simulink model "All_Controller_Compare"  (R2022a)
settings: Solver=VariableStepAuto  StartTime=0.0  StopTime=12.5  RelTol=1e-3
undefined symbols (not defined in the file): A, att_opt, B, C, ki_u4_, Klqr, L, pitch_opt, roll_opt, x_opt, y_opt, yaw_opt
libraries: slpidlib x6
settings Model: Creator=creec  LastModifiedBy=creec

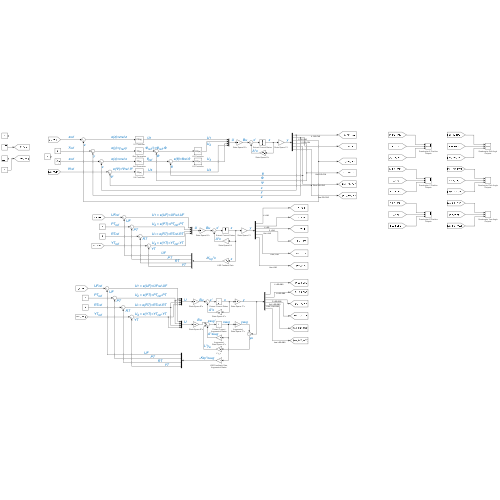
[thumbnail: Simulink's stored preview of the top-level diagram]
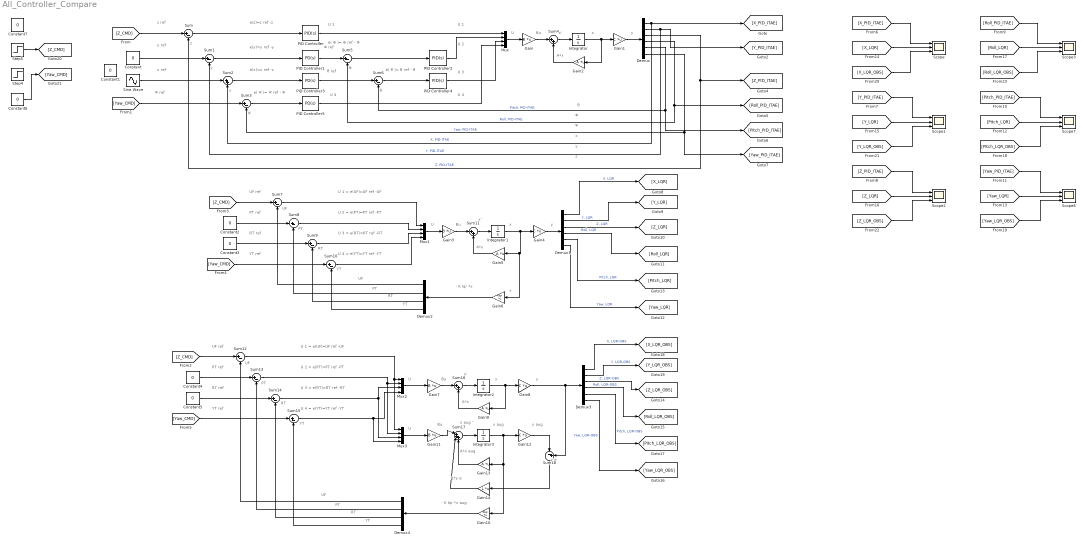
== system All_Controller_Compare ==
  note: z
  note: x ref
  note: U 1
  note: U 4
  note: x
  note: Ψ
  note: x'
  note: θ
  note: Ψ ref
  note: e(y)=y ref -y
  note: e(x)=x ref -x
  note: U 1
  note: e( θ )= θ ref - θ
  note: Φ ref
  note: x
  note: x
  note: Ψ
  note: A*x
  note: e(z)=z ref -z
  note: y
  note: U 2
  note: U
  note: z
  note: θ
  note: Bu
  note: U 4
  note: Φ
  note: Φ
  note: y ref
  note: y
  note: y
  note: z ref
  note: e( Ψ )= Ψ ref - Ψ
  note: U 3
  note: θ ref
  note: e( Φ )= Φ ref - Φ
  note: PT
  note: y
  note: U 3 = e(RT)=RT ref -RT
  note: U 4 = e(YT)=YT ref -YT
  note: U 2 = e(PT)=PT ref -PT
  note: x
  note: RT
  note: PT
  note: - K lqr *x
  note: UF
  note: Bu
  note: UF ref
  note: U 1 = e(UF)=UF ref -UF
  note: RT ref
  note: x
  note: UF
  note: A*x
  note: YT ref
  note: PT ref
  note: U
  note: x'
  note: YT
  note: RT
  note: YT
  note: x aug
  note: L*y e
  note: RT ref
  note: YT ref
  note: x
  note: U
  note: YT
  note: U 1 = e(UF)=UF ref -UF
  note: x'
  note: A*x
  note: YT
  note: A*x aug
  note: PT ref
  note: UF
  note: U
  note: UF
  note: UF ref
  note: Bu
  note: RT
  note: U 2 = e(PT)=PT ref -PT
  note: RT
  note: U 4 = e(YT)=YT ref -YT
  note: x aug '
  note: PT
  note: U 3 = e(RT)=RT ref -RT
  note: PT
  note: y e
  note: - K lqr *x aug
  note: y
  note: y aug
  note: Bu
  Constant{,1..7} (8 alike) : Constant  Value=0
  Demux : Demux  Outputs=6
  Demux1 : Demux  Outputs=6
  Demux2 : Demux
  Demux3 : Demux  Outputs=6
  Demux4 : Demux
  Gain{,3,7,11} (4 alike) : Gain  Gain=B  Multiplication=Matrix(K*u)
      settings: AttributesFormatString=State-Space B*u
  Gain{1,4,8,12} (4 alike) : Gain  Gain=C  Multiplication=Matrix(K*u)
      Gain1 settings: AttributesFormatString=State-Space C*x
      Gain12 settings: AttributesFormatString=|
      | Augmented
      | State-Space C*x
      Gain4 settings: AttributesFormatString=State-Space C*x
      Gain8 settings: AttributesFormatString=State-Space C*x
  Gain10 : Gain  Gain=Klqr  Multiplication=Matrix(K*u)
      settings: AttributesFormatString=|
      | LQR Feedback Gain,
      | Augmented States
  Gain{2,5,9,13} (4 alike) : Gain  Gain=A  Multiplication=Matrix(K*u)
      Gain13 settings: AttributesFormatString=|
      | Augmented
      | State-Space A*x
      Gain2 settings: AttributesFormatString=State-Space A*x
      Gain5 settings: AttributesFormatString=State-Space A*x
      Gain9 settings: AttributesFormatString=State-Space A*x
  Gain14 : Gain  Gain=L  Multiplication=Matrix(K*u)
      settings: AttributesFormatString=L*y_e
  Gain6 : Gain  Gain=Klqr  Multiplication=Matrix(K*u)
      settings: AttributesFormatString=LQR Feeback Gain
  Integrator{,1..3} (4 alike) : Integrator
      Integrator settings: AttributesFormatString=Extract Current States
      Integrator1 settings: AttributesFormatString=Extract Current States
      Integrator2 settings: AttributesFormatString=Extract Current States
      Integrator3 settings: AttributesFormatString=|
      | Extract Current
      | Augmented States
  Mux{,1..3} (4 alike) : Mux
  PID Controller : slpidlib/PID Controller  Controller=PID  Form=Parallel  TimeDomain=Continuous-time  UseExternalTs=off  SampleTime=-1  IntegratorMethod=Forward Euler  FilterMethod=Forward Euler  ControllerParametersSource=internal  P=att_opt(1)  I=att_opt(2)  UseKiTs=off  D=att_opt(3)  N=100  UseFilter=on  TunerSelectOption=Transfer Function Based (PID Tuner App)  InitialConditionSource=internal  InitialConditionForIntegrator=0  InitialConditionForFilter=0  DifferentiatorICPrevScaledInput=0  ExternalReset=none  TrackingMode=off  Kt=1  LimitOutput=off  SatLimitsSource=internal  UpperSaturationLimit=inf  LowerSaturationLimit=-inf  LinearizeAsGain=on  AntiWindupMode=none  Kb=1  POutMin=[]  POutMax=[]  IOutMin=[]  IOutMax=[]  DOutMin=[]  DOutMax=[]  NOutMin=[]  NOutMax=[]  SumOutMin=[]  SumOutMax=[]  SaturationOutMin=[]  SaturationOutMax=[]  PParamMin=[]  PParamMax=[]  IParamMin=[]  IParamMax=[]  DParamMin=[]  DParamMax=[]  NParamMin=[]  NParamMax=[]  KbParamMin=[]  KbParamMax=[]  KtParamMin=[]  KtParamMax=[]  KbOutMin=[]  KbOutMax=[]  KtOutMin=[]  KtOutMax=[]  IntegratorOutMin=[]  IntegratorOutMax=[]  FilterOutMin=[]  FilterOutMax=[]  SumI1OutMin=[]  SumI1OutMax=[]  SumI2OutMin=[]  SumI2OutMax=[]  SumI3OutMin=[]  SumI3OutMax=[]  SumI4OutMin=[]  SumI4OutMax=[]  SumDOutMin=[]  SumDOutMax=[]  DifferentiatorOutMin=[]  DifferentiatorOutMax=[]  FilterDiffOutCoefMin=[]  FilterDiffOutCoefMax=[]  ReciprocalOutMin=[]  ReciprocalOutMax=[]  SumDenOutMin=[]  SumDenOutMax=[]  SumNumOutMin=[]  SumNumOutMax=[]  DivideOutMin=[]  DivideOutMax=[]  UdiffTsProdOutMin=[]  UdiffTsProdOutMax=[]  NTsProdOutMin=[]  NTsProdOutMax=[]  UintegralTsProdOutMin=[]  UintegralTsProdOutMax=[]  UngainTsProdOutMin=[]  UngainTsProdOutMax=[]  IntegratorContinuousStateAttributes=''  IntegratorStateMustResolveToSignalObject=off  IntegratorRTWStateStorageClass=Auto  FilterContinuousStateAttributes=''  FilterStateMustResolveToSignalObject=off  FilterRTWStateStorageClass=Auto  ParallelPVariant=InternalParameters  IdealPVariant=Disabled  IVariant=InternalParameters  DVariant=InternalParameters  IntegratorVariant=Continuous  SatVariant=Disabled  AWVariant=Passthrough  PCopyVariant=Disabled  TRVariant=Disabled  FdbkBlocksVariant=Forward  IdealPFdbkVariant=Disabled  SatFdbkVariant=Disabled  DerivativeFilterVariant=ContFilter  NVariant=InternalParameters  NCopyVariant=Disabled  FilterICVariant=InternalICsFilter  IntegratorICVariant=InternalICs  ExternalResetVariant=Disabled  TRSumVariant=Passthrough  SumFdbkVariant=Disabled  SumVariant=Sum_PID  TsampFilterVariant=InternalTs  TsampNgainVariant=Passthrough  TsampIntegralVariant=Passthrough  ExternalSaturationOutDataTypeStr=Inherit: Same as second input  aMode=0
      settings: AttributesFormatString=U1 Controller
  PID Controller1 : slpidlib/PID Controller  Controller=PD  Form=Parallel  TimeDomain=Continuous-time  UseExternalTs=off  SampleTime=-1  IntegratorMethod=Forward Euler  FilterMethod=Forward Euler  ControllerParametersSource=internal  P=y_opt(1)  I=0  UseKiTs=off  D=y_opt(2)  N=100  UseFilter=on  TunerSelectOption=Transfer Function Based (PID Tuner App)  InitialConditionSource=internal  InitialConditionForIntegrator=0  InitialConditionForFilter=0  DifferentiatorICPrevScaledInput=0  ExternalReset=none  TrackingMode=off  Kt=1  LimitOutput=off  SatLimitsSource=internal  UpperSaturationLimit=inf  LowerSaturationLimit=-inf  LinearizeAsGain=on  AntiWindupMode=none  Kb=1  POutMin=[]  POutMax=[]  IOutMin=[]  IOutMax=[]  DOutMin=[]  DOutMax=[]  NOutMin=[]  NOutMax=[]  SumOutMin=[]  SumOutMax=[]  SaturationOutMin=[]  SaturationOutMax=[]  PParamMin=[]  PParamMax=[]  IParamMin=[]  IParamMax=[]  DParamMin=[]  DParamMax=[]  NParamMin=[]  NParamMax=[]  KbParamMin=[]  KbParamMax=[]  KtParamMin=[]  KtParamMax=[]  KbOutMin=[]  KbOutMax=[]  KtOutMin=[]  KtOutMax=[]  IntegratorOutMin=[]  IntegratorOutMax=[]  FilterOutMin=[]  FilterOutMax=[]  SumI1OutMin=[]  SumI1OutMax=[]  SumI2OutMin=[]  SumI2OutMax=[]  SumI3OutMin=[]  SumI3OutMax=[]  SumI4OutMin=[]  SumI4OutMax=[]  SumDOutMin=[]  SumDOutMax=[]  DifferentiatorOutMin=[]  DifferentiatorOutMax=[]  FilterDiffOutCoefMin=[]  FilterDiffOutCoefMax=[]  ReciprocalOutMin=[]  ReciprocalOutMax=[]  SumDenOutMin=[]  SumDenOutMax=[]  SumNumOutMin=[]  SumNumOutMax=[]  DivideOutMin=[]  DivideOutMax=[]  UdiffTsProdOutMin=[]  UdiffTsProdOutMax=[]  NTsProdOutMin=[]  NTsProdOutMax=[]  UintegralTsProdOutMin=[]  UintegralTsProdOutMax=[]  UngainTsProdOutMin=[]  UngainTsProdOutMax=[]  IntegratorContinuousStateAttributes=''  IntegratorStateMustResolveToSignalObject=off  IntegratorRTWStateStorageClass=Auto  FilterContinuousStateAttributes=''  FilterStateMustResolveToSignalObject=off  FilterRTWStateStorageClass=Auto  ParallelPVariant=InternalParameters  IdealPVariant=Disabled  IVariant=Disabled  DVariant=InternalParameters  IntegratorVariant=Disabled  SatVariant=Disabled  AWVariant=Disabled  PCopyVariant=Disabled  TRVariant=Disabled  FdbkBlocksVariant=Forward  IdealPFdbkVariant=Disabled  SatFdbkVariant=Disabled  DerivativeFilterVariant=ContFilter  NVariant=InternalParameters  NCopyVariant=Disabled  FilterICVariant=InternalICsFilter  IntegratorICVariant=Disabled  ExternalResetVariant=Disabled  TRSumVariant=Passthrough  SumFdbkVariant=Disabled  SumVariant=Sum_PD  TsampFilterVariant=InternalTs  TsampNgainVariant=Passthrough  TsampIntegralVariant=Disabled_SignalSpec  ExternalSaturationOutDataTypeStr=Inherit: Same as second input  aMode=0
      settings: AttributesFormatString=Φref Generation
  PID Controller2 : slpidlib/PID Controller  Controller=PID  Form=Parallel  TimeDomain=Continuous-time  UseExternalTs=off  SampleTime=-1  IntegratorMethod=Forward Euler  FilterMethod=Forward Euler  ControllerParametersSource=internal  P=pitch_opt(1)  I=pitch_opt(2)  UseKiTs=off  D=pitch_opt(3)  N=100  UseFilter=on  TunerSelectOption=Transfer Function Based (PID Tuner App)  InitialConditionSource=internal  InitialConditionForIntegrator=0  InitialConditionForFilter=0  DifferentiatorICPrevScaledInput=0  ExternalReset=none  TrackingMode=off  Kt=1  LimitOutput=off  SatLimitsSource=internal  UpperSaturationLimit=inf  LowerSaturationLimit=-inf  LinearizeAsGain=on  AntiWindupMode=none  Kb=1  POutMin=[]  POutMax=[]  IOutMin=[]  IOutMax=[]  DOutMin=[]  DOutMax=[]  NOutMin=[]  NOutMax=[]  SumOutMin=[]  SumOutMax=[]  SaturationOutMin=[]  SaturationOutMax=[]  PParamMin=[]  PParamMax=[]  IParamMin=[]  IParamMax=[]  DParamMin=[]  DParamMax=[]  NParamMin=[]  NParamMax=[]  KbParamMin=[]  KbParamMax=[]  KtParamMin=[]  KtParamMax=[]  KbOutMin=[]  KbOutMax=[]  KtOutMin=[]  KtOutMax=[]  IntegratorOutMin=[]  IntegratorOutMax=[]  FilterOutMin=[]  FilterOutMax=[]  SumI1OutMin=[]  SumI1OutMax=[]  SumI2OutMin=[]  SumI2OutMax=[]  SumI3OutMin=[]  SumI3OutMax=[]  SumI4OutMin=[]  SumI4OutMax=[]  SumDOutMin=[]  SumDOutMax=[]  DifferentiatorOutMin=[]  DifferentiatorOutMax=[]  FilterDiffOutCoefMin=[]  FilterDiffOutCoefMax=[]  ReciprocalOutMin=[]  ReciprocalOutMax=[]  SumDenOutMin=[]  SumDenOutMax=[]  SumNumOutMin=[]  SumNumOutMax=[]  DivideOutMin=[]  DivideOutMax=[]  UdiffTsProdOutMin=[]  UdiffTsProdOutMax=[]  NTsProdOutMin=[]  NTsProdOutMax=[]  UintegralTsProdOutMin=[]  UintegralTsProdOutMax=[]  UngainTsProdOutMin=[]  UngainTsProdOutMax=[]  IntegratorContinuousStateAttributes=''  IntegratorStateMustResolveToSignalObject=off  IntegratorRTWStateStorageClass=Auto  FilterContinuousStateAttributes=''  FilterStateMustResolveToSignalObject=off  FilterRTWStateStorageClass=Auto  ParallelPVariant=InternalParameters  IdealPVariant=Disabled  IVariant=InternalParameters  DVariant=InternalParameters  IntegratorVariant=Continuous  SatVariant=Disabled  AWVariant=Passthrough  PCopyVariant=Disabled  TRVariant=Disabled  FdbkBlocksVariant=Forward  IdealPFdbkVariant=Disabled  SatFdbkVariant=Disabled  DerivativeFilterVariant=ContFilter  NVariant=InternalParameters  NCopyVariant=Disabled  FilterICVariant=InternalICsFilter  IntegratorICVariant=InternalICs  ExternalResetVariant=Disabled  TRSumVariant=Passthrough  SumFdbkVariant=Disabled  SumVariant=Sum_PID  TsampFilterVariant=InternalTs  TsampNgainVariant=Passthrough  TsampIntegralVariant=Passthrough  ExternalSaturationOutDataTypeStr=Inherit: Same as second input  aMode=0
      settings: AttributesFormatString=U2 Controller
  PID Controller3 : slpidlib/PID Controller  Controller=PD  Form=Parallel  TimeDomain=Continuous-time  UseExternalTs=off  SampleTime=-1  IntegratorMethod=Forward Euler  FilterMethod=Forward Euler  ControllerParametersSource=internal  P=x_opt(1)  I=-0.0096  UseKiTs=off  D=x_opt(2)  N=100  UseFilter=on  TunerSelectOption=Transfer Function Based (PID Tuner App)  InitialConditionSource=internal  InitialConditionForIntegrator=0  InitialConditionForFilter=0  DifferentiatorICPrevScaledInput=0  ExternalReset=none  TrackingMode=off  Kt=1  LimitOutput=off  SatLimitsSource=internal  UpperSaturationLimit=inf  LowerSaturationLimit=-inf  LinearizeAsGain=on  AntiWindupMode=none  Kb=1  POutMin=[]  POutMax=[]  IOutMin=[]  IOutMax=[]  DOutMin=[]  DOutMax=[]  NOutMin=[]  NOutMax=[]  SumOutMin=[]  SumOutMax=[]  SaturationOutMin=[]  SaturationOutMax=[]  PParamMin=[]  PParamMax=[]  IParamMin=[]  IParamMax=[]  DParamMin=[]  DParamMax=[]  NParamMin=[]  NParamMax=[]  KbParamMin=[]  KbParamMax=[]  KtParamMin=[]  KtParamMax=[]  KbOutMin=[]  KbOutMax=[]  KtOutMin=[]  KtOutMax=[]  IntegratorOutMin=[]  IntegratorOutMax=[]  FilterOutMin=[]  FilterOutMax=[]  SumI1OutMin=[]  SumI1OutMax=[]  SumI2OutMin=[]  SumI2OutMax=[]  SumI3OutMin=[]  SumI3OutMax=[]  SumI4OutMin=[]  SumI4OutMax=[]  SumDOutMin=[]  SumDOutMax=[]  DifferentiatorOutMin=[]  DifferentiatorOutMax=[]  FilterDiffOutCoefMin=[]  FilterDiffOutCoefMax=[]  ReciprocalOutMin=[]  ReciprocalOutMax=[]  SumDenOutMin=[]  SumDenOutMax=[]  SumNumOutMin=[]  SumNumOutMax=[]  DivideOutMin=[]  DivideOutMax=[]  UdiffTsProdOutMin=[]  UdiffTsProdOutMax=[]  NTsProdOutMin=[]  NTsProdOutMax=[]  UintegralTsProdOutMin=[]  UintegralTsProdOutMax=[]  UngainTsProdOutMin=[]  UngainTsProdOutMax=[]  IntegratorContinuousStateAttributes=''  IntegratorStateMustResolveToSignalObject=off  IntegratorRTWStateStorageClass=Auto  FilterContinuousStateAttributes=''  FilterStateMustResolveToSignalObject=off  FilterRTWStateStorageClass=Auto  ParallelPVariant=InternalParameters  IdealPVariant=Disabled  IVariant=Disabled  DVariant=InternalParameters  IntegratorVariant=Disabled  SatVariant=Disabled  AWVariant=Disabled  PCopyVariant=Disabled  TRVariant=Disabled  FdbkBlocksVariant=Forward  IdealPFdbkVariant=Disabled  SatFdbkVariant=Disabled  DerivativeFilterVariant=ContFilter  NVariant=InternalParameters  NCopyVariant=Disabled  FilterICVariant=InternalICsFilter  IntegratorICVariant=Disabled  ExternalResetVariant=Disabled  TRSumVariant=Passthrough  SumFdbkVariant=Disabled  SumVariant=Sum_PD  TsampFilterVariant=InternalTs  TsampNgainVariant=Passthrough  TsampIntegralVariant=Disabled_SignalSpec  ExternalSaturationOutDataTypeStr=Inherit: Same as second input  aMode=0
      settings: AttributesFormatString=θref Generation
  PID Controller4 : slpidlib/PID Controller  Controller=PID  Form=Parallel  TimeDomain=Continuous-time  UseExternalTs=off  SampleTime=-1  IntegratorMethod=Forward Euler  FilterMethod=Forward Euler  ControllerParametersSource=internal  P=roll_opt(1)  I=roll_opt(2)  UseKiTs=off  D=roll_opt(3)  N=100  UseFilter=on  TunerSelectOption=Transfer Function Based (PID Tuner App)  InitialConditionSource=internal  InitialConditionForIntegrator=0  InitialConditionForFilter=0  DifferentiatorICPrevScaledInput=0  ExternalReset=none  TrackingMode=off  Kt=1  LimitOutput=off  SatLimitsSource=internal  UpperSaturationLimit=inf  LowerSaturationLimit=-inf  LinearizeAsGain=on  AntiWindupMode=none  Kb=1  POutMin=[]  POutMax=[]  IOutMin=[]  IOutMax=[]  DOutMin=[]  DOutMax=[]  NOutMin=[]  NOutMax=[]  SumOutMin=[]  SumOutMax=[]  SaturationOutMin=[]  SaturationOutMax=[]  PParamMin=[]  PParamMax=[]  IParamMin=[]  IParamMax=[]  DParamMin=[]  DParamMax=[]  NParamMin=[]  NParamMax=[]  KbParamMin=[]  KbParamMax=[]  KtParamMin=[]  KtParamMax=[]  KbOutMin=[]  KbOutMax=[]  KtOutMin=[]  KtOutMax=[]  IntegratorOutMin=[]  IntegratorOutMax=[]  FilterOutMin=[]  FilterOutMax=[]  SumI1OutMin=[]  SumI1OutMax=[]  SumI2OutMin=[]  SumI2OutMax=[]  SumI3OutMin=[]  SumI3OutMax=[]  SumI4OutMin=[]  SumI4OutMax=[]  SumDOutMin=[]  SumDOutMax=[]  DifferentiatorOutMin=[]  DifferentiatorOutMax=[]  FilterDiffOutCoefMin=[]  FilterDiffOutCoefMax=[]  ReciprocalOutMin=[]  ReciprocalOutMax=[]  SumDenOutMin=[]  SumDenOutMax=[]  SumNumOutMin=[]  SumNumOutMax=[]  DivideOutMin=[]  DivideOutMax=[]  UdiffTsProdOutMin=[]  UdiffTsProdOutMax=[]  NTsProdOutMin=[]  NTsProdOutMax=[]  UintegralTsProdOutMin=[]  UintegralTsProdOutMax=[]  UngainTsProdOutMin=[]  UngainTsProdOutMax=[]  IntegratorContinuousStateAttributes=''  IntegratorStateMustResolveToSignalObject=off  IntegratorRTWStateStorageClass=Auto  FilterContinuousStateAttributes=''  FilterStateMustResolveToSignalObject=off  FilterRTWStateStorageClass=Auto  ParallelPVariant=InternalParameters  IdealPVariant=Disabled  IVariant=InternalParameters  DVariant=InternalParameters  IntegratorVariant=Continuous  SatVariant=Disabled  AWVariant=Passthrough  PCopyVariant=Disabled  TRVariant=Disabled  FdbkBlocksVariant=Forward  IdealPFdbkVariant=Disabled  SatFdbkVariant=Disabled  DerivativeFilterVariant=ContFilter  NVariant=InternalParameters  NCopyVariant=Disabled  FilterICVariant=InternalICsFilter  IntegratorICVariant=InternalICs  ExternalResetVariant=Disabled  TRSumVariant=Passthrough  SumFdbkVariant=Disabled  SumVariant=Sum_PID  TsampFilterVariant=InternalTs  TsampNgainVariant=Passthrough  TsampIntegralVariant=Passthrough  ExternalSaturationOutDataTypeStr=Inherit: Same as second input  aMode=0
      settings: AttributesFormatString=U3 Controller
  PID Controller5 : slpidlib/PID Controller  Controller=PD  Form=Parallel  TimeDomain=Continuous-time  UseExternalTs=off  SampleTime=-1  IntegratorMethod=Forward Euler  FilterMethod=Forward Euler  ControllerParametersSource=internal  P=yaw_opt(1)  I=ki_u4_  UseKiTs=off  D=yaw_opt(2)  N=100  UseFilter=on  TunerSelectOption=Transfer Function Based (PID Tuner App)  InitialConditionSource=internal  InitialConditionForIntegrator=0  InitialConditionForFilter=0  DifferentiatorICPrevScaledInput=0  ExternalReset=none  TrackingMode=off  Kt=1  LimitOutput=off  SatLimitsSource=internal  UpperSaturationLimit=inf  LowerSaturationLimit=-inf  LinearizeAsGain=on  AntiWindupMode=none  Kb=1  POutMin=[]  POutMax=[]  IOutMin=[]  IOutMax=[]  DOutMin=[]  DOutMax=[]  NOutMin=[]  NOutMax=[]  SumOutMin=[]  SumOutMax=[]  SaturationOutMin=[]  SaturationOutMax=[]  PParamMin=[]  PParamMax=[]  IParamMin=[]  IParamMax=[]  DParamMin=[]  DParamMax=[]  NParamMin=[]  NParamMax=[]  KbParamMin=[]  KbParamMax=[]  KtParamMin=[]  KtParamMax=[]  KbOutMin=[]  KbOutMax=[]  KtOutMin=[]  KtOutMax=[]  IntegratorOutMin=[]  IntegratorOutMax=[]  FilterOutMin=[]  FilterOutMax=[]  SumI1OutMin=[]  SumI1OutMax=[]  SumI2OutMin=[]  SumI2OutMax=[]  SumI3OutMin=[]  SumI3OutMax=[]  SumI4OutMin=[]  SumI4OutMax=[]  SumDOutMin=[]  SumDOutMax=[]  DifferentiatorOutMin=[]  DifferentiatorOutMax=[]  FilterDiffOutCoefMin=[]  FilterDiffOutCoefMax=[]  ReciprocalOutMin=[]  ReciprocalOutMax=[]  SumDenOutMin=[]  SumDenOutMax=[]  SumNumOutMin=[]  SumNumOutMax=[]  DivideOutMin=[]  DivideOutMax=[]  UdiffTsProdOutMin=[]  UdiffTsProdOutMax=[]  NTsProdOutMin=[]  NTsProdOutMax=[]  UintegralTsProdOutMin=[]  UintegralTsProdOutMax=[]  UngainTsProdOutMin=[]  UngainTsProdOutMax=[]  IntegratorContinuousStateAttributes=''  IntegratorStateMustResolveToSignalObject=off  IntegratorRTWStateStorageClass=Auto  FilterContinuousStateAttributes=''  FilterStateMustResolveToSignalObject=off  FilterRTWStateStorageClass=Auto  ParallelPVariant=InternalParameters  IdealPVariant=Disabled  IVariant=Disabled  DVariant=InternalParameters  IntegratorVariant=Disabled  SatVariant=Disabled  AWVariant=Disabled  PCopyVariant=Disabled  TRVariant=Disabled  FdbkBlocksVariant=Forward  IdealPFdbkVariant=Disabled  SatFdbkVariant=Disabled  DerivativeFilterVariant=ContFilter  NVariant=InternalParameters  NCopyVariant=Disabled  FilterICVariant=InternalICsFilter  IntegratorICVariant=Disabled  ExternalResetVariant=Disabled  TRSumVariant=Passthrough  SumFdbkVariant=Disabled  SumVariant=Sum_PD  TsampFilterVariant=InternalTs  TsampNgainVariant=Passthrough  TsampIntegralVariant=Disabled_SignalSpec  ExternalSaturationOutDataTypeStr=Inherit: Same as second input  aMode=0
      settings: AttributesFormatString=U4 Controller
  Scope{,1..3,7..8} (6 alike) : Scope  NumInputPorts=3
      Scope settings: AttributesFormatString=|
      | Quadcopter X-Position
      | Outputs
      Scope1 settings: AttributesFormatString=|
      | Quadcopter Y-Position
      | Outputs
      Scope2 settings: AttributesFormatString=|
      | Quadcopter Z-Position
      | Outputs
      Scope3 settings: AttributesFormatString=|
      | Quadcopter Roll Angle
      | Outputs
      Scope7 settings: AttributesFormatString=|
      | Quadcopter Pitch Angle
      | Outputs
      Scope8 settings: AttributesFormatString=|
      | Quadcopter Yaw Angle
      | Outputs
  Sine Wave : Sin  Amplitude=20  Frequency=0.3142  SampleTime=0
  Step4 : Step  Time=0  After=5  SampleTime=0
  Step5 : Step  After=8  SampleTime=0
  Sum{,1,3,5..10,12..15} (13 alike) : Sum  Inputs=|+-
  Sum{2,4,11,16} (4 alike) : Sum  Inputs=|++
  Sum17 : Sum  Inputs=|+++
  Sum18 : Sum  Inputs=|-+
  wires:
  Demux/1 -> [X_PID_ITAE], Sum2/2  "X, PID-ITAE"
  Demux/2 -> [Y_PID_ITAE], Sum1/2  "Y, PID-ITAE"
  Constant/1 -> Sum1/1
  Demux/5 -> [Pitch_PID_ITAE], Sum6/2  "Pitch, PID-ITAE"
  Sine Wave/1 -> Sum2/1
  PID Controller5/1 -> Mux/4
  [Yaw_CMD] -> Sum3/1
  Sum6/1 -> PID Controller4/1
  PID Controller3/1 -> Sum6/1
  [Z_CMD] -> Sum/1
  PID Controller/1 -> Mux/1
  Mux/1 -> Gain/1
  Demux/4 -> [Roll_PID_ITAE], Sum5/2  "Roll, PID-ITAE"
  Demux/3 -> [Z_PID_ITAE], Sum/2  "Z, PID-ITAE"
  Demux/6 -> [Yaw_PID_ITAE], Sum3/2  "Yaw, PID-ITAE"
  Sum5/1 -> PID Controller2/1
  Integrator/1 -> Gain2/1, Gain1/1
  Sum2/1 -> PID Controller3/1
  Sum1/1 -> PID Controller1/1
  PID Controller1/1 -> Sum5/1
  Sum4/1 -> Integrator/1
  Sum/1 -> PID Controller/1
  PID Controller4/1 -> Mux/3
  Gain2/1 -> Sum4/2
  PID Controller2/1 -> Mux/2
  Sum3/1 -> PID Controller5/1
  Gain/1 -> Sum4/1
  Gain1/1 -> Demux/1
  Gain4/1 -> Demux1/1
  Sum8/1 -> Mux1/2
  Demux2/3 -> Sum9/2
  Sum9/1 -> Mux1/3
  Demux2/2 -> Sum8/2
  Demux1/5 -> [Pitch_LQR]  "Pitch, LQR"
  Constant2/1 -> Sum8/1
  Constant3/1 -> Sum9/1
  Gain6/1 -> Demux2/1
  Demux1/6 -> [Yaw_LQR]  "Yaw, LQR"
  [Yaw_CMD] -> Sum10/1
  Gain3/1 -> Sum11/1
  Demux2/1 -> Sum7/2
  Sum10/1 -> Mux1/4
  Demux1/1 -> [X_LQR]  "X, LQR"
  Demux1/3 -> [Z_LQR]  "Z, LQR"
  Gain5/1 -> Sum11/2
  Demux1/4 -> [Roll_LQR]  "Roll, LQR"
  Integrator1/1 -> Gain4/1, Gain6/1, Gain5/1
  Mux1/1 -> Gain3/1
  Demux1/2 -> [Y_LQR]  "Y, LQR"
  Demux2/4 -> Sum10/2
  [Z_CMD] -> Sum7/1
  Sum7/1 -> Mux1/1
  Sum11/1 -> Integrator1/1
  Gain14/1 -> Sum17/2
  Integrator3/1 -> Gain10/1, Gain13/1, Gain12/1
  Sum17/1 -> Integrator3/1
  Demux4/4 -> Sum15/2
  [Z_CMD] -> Sum12/1
  Sum12/1 -> Mux3/1, Mux2/1
  Gain11/1 -> Sum17/1
  Integrator2/1 -> Gain9/1, Gain8/1
  Mux2/1 -> Gain7/1
  Sum16/1 -> Integrator2/1
  Demux4/2 -> Sum13/2
  [Yaw_CMD] -> Sum15/1
  Gain9/1 -> Sum16/2
  Gain7/1 -> Sum16/1
  Demux3/5 -> [Pitch_LQR_OBS]  "Pitch, LQR-OBS"
  Sum15/1 -> Mux2/4, Mux3/4
  Constant4/1 -> Sum13/1
  Demux4/1 -> Sum12/2
  Sum14/1 -> Mux2/3, Mux3/3
  Demux4/3 -> Sum14/2
  Gain8/1 -> Sum18/2, Demux3/1
  Sum13/1 -> Mux2/2, Mux3/2
  Constant5/1 -> Sum14/1
  Gain13/1 -> Sum17/3
  Mux3/1 -> Gain11/1
  Sum18/1 -> Gain14/1
  Gain10/1 -> Demux4/1
  Demux3/4 -> [Roll_LQR_OBS]  "Roll, LQR-OBS"
  Demux3/3 -> [Z_LQR_OBS]  "Z, LQR-OBS"
  Demux3/2 -> [Y_LQR_OBS]  "Y, LQR-OBS"
  Demux3/6 -> [Yaw_LQR_OBS]  "Yaw, LQR-OBS"
  Gain12/1 -> Sum18/1
  Demux3/1 -> [X_LQR_OBS]  "X, LQR-OBS"
  [X_PID_ITAE] -> Scope/1
  [X_LQR] -> Scope/2
  [X_LQR_OBS] -> Scope/3
  [Y_LQR] -> Scope1/2
  [Y_PID_ITAE] -> Scope1/1
  [Y_LQR_OBS] -> Scope1/3
  [Z_PID_ITAE] -> Scope2/1
  [Z_LQR] -> Scope2/2
  [Z_LQR_OBS] -> Scope2/3
  [Yaw_PID_ITAE] -> Scope8/1
  [Roll_LQR_OBS] -> Scope3/3
  [Pitch_PID_ITAE] -> Scope7/1
  [Roll_LQR] -> Scope3/2
  [Yaw_LQR] -> Scope8/2
  [Pitch_LQR] -> Scope7/2
  [Yaw_LQR_OBS] -> Scope8/3
  [Pitch_LQR_OBS] -> Scope7/3
  [Roll_PID_ITAE] -> Scope3/1
  Step5/1 -> [Z_CMD]
  Constant6/1 -> [Yaw_CMD]
